simulink model "pt2_signal3_saturation"  (R2019a)
settings: Solver=ode4  StartTime=0.0  StopTime=0.1  FixedStep=1e-4  RelTol=1e-3
settings Model: Creator=guima  LastModifiedBy=guima

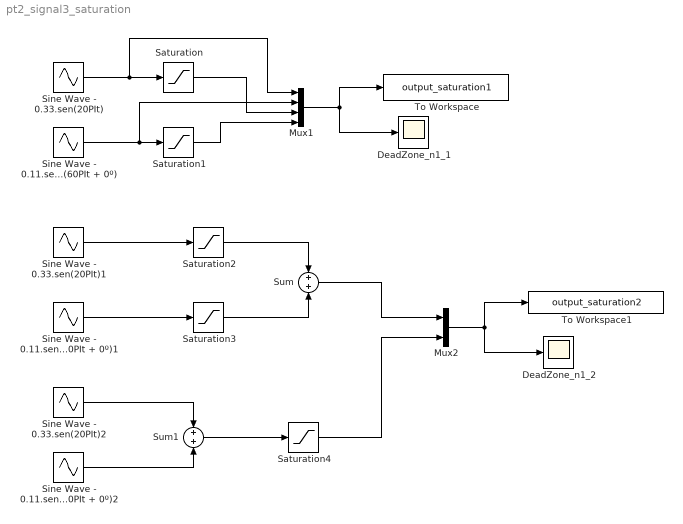
== system pt2_signal3_saturation ==
  "DeadZone_n1_1 " : Scope
  DeadZone_n1_2 : Scope
  Mux1 : Mux
  Mux2 : Mux  Inputs=2
  Saturation{,1..4} (5 alike) : Saturate  UpperLimit=0.1  LowerLimit=-0.1
  Sine Wave - 0.11.sen(60PIt + 0º) : Sin  Amplitude=0.11  Frequency=60*pi  SampleTime=0
  Sine Wave - 0.11.sen(60PIt + 0º)1 : Sin  Amplitude=0.11  Frequency=60*pi  SampleTime=0
  Sine Wave - 0.11.sen(60PIt + 0º)2 : Sin  Amplitude=0.11  Frequency=60*pi  SampleTime=0
  Sine Wave - 0.33.sen(20PIt) : Sin  Amplitude=0.33  Frequency=20*pi  SampleTime=0
  Sine Wave - 0.33.sen(20PIt)1 : Sin  Amplitude=0.33  Frequency=20*pi  SampleTime=0
  Sine Wave - 0.33.sen(20PIt)2 : Sin  Amplitude=0.33  Frequency=20*pi  SampleTime=0
  Sum : Sum
  Sum1 : Sum
  To Workspace : ToWorkspace  VariableName=output_saturation1  SaveFormat=Structure With Time  SampleTime=-1
  To Workspace1 : ToWorkspace  VariableName=output_saturation2  SaveFormat=Structure With Time  SampleTime=-1
  wires:
  Mux1/1 -> "DeadZone_n1_1 "/1, To Workspace/1
  Sine Wave - 0.11.sen(60PIt + 0º)/1 -> Mux1/2, Saturation1/1
  Sine Wave - 0.33.sen(20PIt)/1 -> Mux1/1, Saturation/1
  Sine Wave - 0.33.sen(20PIt)1/1 -> Saturation2/1
  Mux2/1 -> DeadZone_n1_2/1, To Workspace1/1
  Sine Wave - 0.11.sen(60PIt + 0º)1/1 -> Saturation3/1
  Sum/1 -> Mux2/1
  Sine Wave - 0.33.sen(20PIt)2/1 -> Sum1/1
  Sine Wave - 0.11.sen(60PIt + 0º)2/1 -> Sum1/2
  Sum1/1 -> Saturation4/1
  Saturation4/1 -> Mux2/2
  Saturation2/1 -> Sum/1
  Saturation3/1 -> Sum/2
  Saturation/1 -> Mux1/3
  Saturation1/1 -> Mux1/4
